simulink model "sampleModel261"  (R2021b)
settings: Solver=VariableStepAuto  StartTime=0.0  StopTime=10.0  RelTol=1e-3
undefined symbols (not defined in the file or in its folder): DiscIntNeverNeededParam
libraries: simulink x6, slpidlib x2
settings Model: Creator=user  LastModifiedBy=user

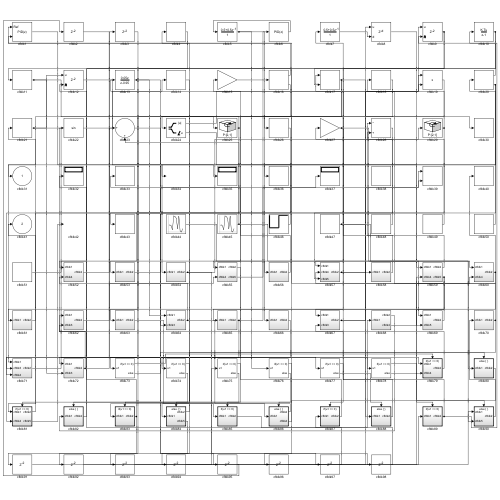
[thumbnail: Simulink's stored preview of the top-level diagram]
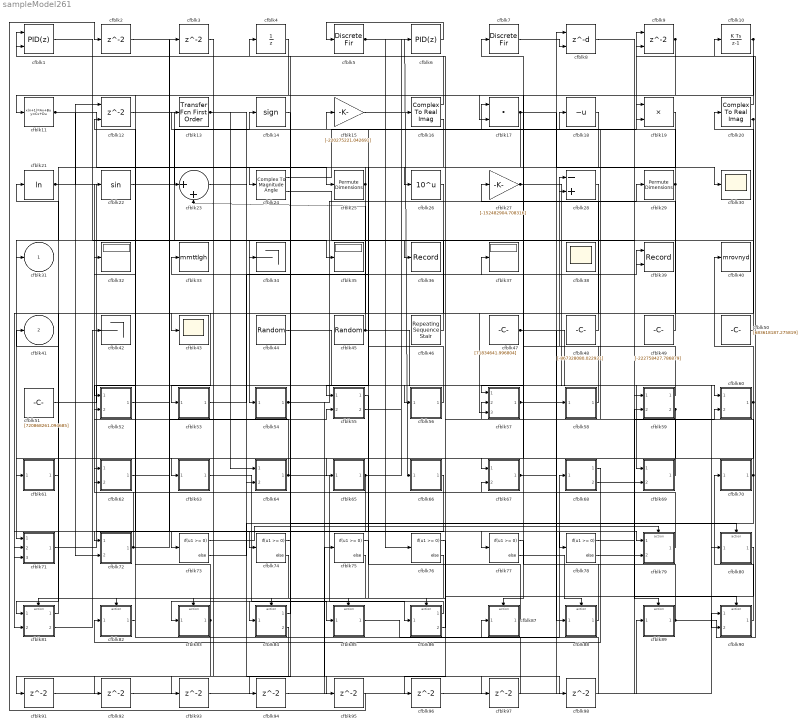
== system sampleModel261 ==
  cfblk1 : slpidlib/PID Controller (2DOF)  Controller=PID  Form=Parallel  TimeDomain=Discrete-time  UseExternalTs=off  SampleTime=1  IntegratorMethod=Forward Euler  FilterMethod=Forward Euler  ControllerParametersSource=internal  P=1  I=1  D=0  UseFilter=on  N=100  b=1  c=1  TunerSelectOption=Transfer Function Based (PID Tuner App)  InitialConditionSource=internal  InitialConditionForIntegrator=0  InitialConditionForFilter=0  DifferentiatorICPrevScaledInput=0  ExternalReset=none  TrackingMode=off  Kt=1  LimitOutput=off  SatLimitsSource=internal  UpperSaturationLimit=inf  LowerSaturationLimit=-inf  LinearizeAsGain=off  AntiWindupMode=none  Kb=1  POutMin=[]  POutMax=[]  IOutMin=[]  IOutMax=[]  DOutMin=[]  DOutMax=[]  NOutMin=[]  NOutMax=[]  bOutMin=[]  bOutMax=[]  cOutMin=[]  cOutMax=[]  SumOutMin=[]  SumOutMax=[]  SaturationOutMin=[]  SaturationOutMax=[]  PParamMin=[]  PParamMax=[]  IParamMin=[]  IParamMax=[]  DParamMin=[]  DParamMax=[]  NParamMin=[]  NParamMax=[]  bParamMin=[]  bParamMax=[]  cParamMin=[]  cParamMax=[]  KbParamMin=[]  KbParamMax=[]  KtParamMin=[]  KtParamMax=[]  KbOutMin=[]  KbOutMax=[]  KtOutMin=[]  KtOutMax=[]  IntegratorOutMin=[]  IntegratorOutMax=[]  FilterOutMin=[]  FilterOutMax=[]  SumI1OutMin=[]  SumI1OutMax=[]  SumI2OutMin=[]  SumI2OutMax=[]  SumI3OutMin=[]  SumI3OutMax=[]  SumI4OutMin=[]  SumI4OutMax=[]  SumDOutMin=[]  SumDOutMax=[]  Sum1OutMin=[]  Sum1OutMax=[]  Sum2OutMin=[]  Sum2OutMax=[]  Sum3OutMin=[]  Sum3OutMax=[]  DifferentiatorOutMin=[]  DifferentiatorOutMax=[]  FilterDiffOutCoefMin=[]  FilterDiffOutCoefMax=[]  ReciprocalOutMin=[]  ReciprocalOutMax=[]  SumDenOutMin=[]  SumDenOutMax=[]  SumNumOutMin=[]  SumNumOutMax=[]  DivideOutMin=[]  DivideOutMax=[]  UdiffTsProdOutMin=[]  UdiffTsProdOutMax=[]  NTsProdOutMin=[]  NTsProdOutMax=[]  UintegralTsProdOutMin=[]  UintegralTsProdOutMax=[]  UngainTsProdOutMin=[]  UngainTsProdOutMax=[]  IntegratorContinuousStateAttributes=''  IntegratorStateMustResolveToSignalObject=off  IntegratorRTWStateStorageClass=Auto  FilterContinuousStateAttributes=''  FilterStateMustResolveToSignalObject=off  FilterRTWStateStorageClass=Auto  ParallelPVariant=InternalParameters  IdealPVariant=Disabled  IVariant=InternalParameters  DVariant=InternalParameters  bVariant=InternalParameters  cVariant=InternalParameters  IntegratorVariant=Discrete  SatVariant=Disabled  AWVariant=Passthrough  PCopyVariant=Disabled  TRVariant=Disabled  FdbkBlocksVariant=Forward  IdealPFdbkVariant=Disabled  SatFdbkVariant=Disabled  DerivativeFilterVariant=ForwardEulerFilter  NVariant=InternalParameters  NCopyVariant=Disabled  FilterICVariant=InternalICsFilter  IntegratorICVariant=InternalICs  ExternalResetVariant=Disabled  TRSumVariant=Passthrough  SumFdbkVariant=Disabled  SumVariant=Sum_PID  TsampFilterVariant=InternalTs  TsampNgainVariant=Passthrough  TsampIntegralVariant=Passthrough  ExternalSaturationOutDataTypeStr=Inherit: Same as second input
      settings: SourceProductBaseCode=SL
  cfblk10 : DiscreteIntegrator  ICPrevOutput=DiscIntNeverNeededParam  ICPrevScaledInput=DiscIntNeverNeededParam
  cfblk11 : DiscreteStateSpace
  cfblk12 : Delay  ShowEnablePort=on  SampleTime=1
      settings: InputPortMap=u0,e6
  cfblk13 : simulink/Discrete/Transfer Fcn First Order  PoleZ=0.95  ICPrevOutput=0.0  DoSatur=off
  cfblk14 : Signum
  cfblk15 : Gain  Gain=[-220275221.042691]
  cfblk16 : ComplexToRealImag
  cfblk17 : DotProduct  InputSameDT=on  OutDataTypeStr=Inherit: Inherit via internal rule
  cfblk18 : UnaryMinus
  cfblk19 : Product
  cfblk{2..3,91..98} (10 alike) : Delay  SampleTime=1
  cfblk20 : ComplexToRealImag
  cfblk21 : Math  Operator=log  SaturateOnIntegerOverflow=on
  cfblk22 : Trigonometry
  cfblk23 : Sum  Inputs=|++
  cfblk24 : ComplexToMagnitudeAngle
  cfblk25 : PermuteDimensions
  cfblk26 : Math  Operator=10^u  SaturateOnIntegerOverflow=on
  cfblk27 : Gain  Gain=[-152482904.708316]
  cfblk28 : Sum  Inputs=-+
  cfblk29 : PermuteDimensions
  cfblk30 : Scope
  cfblk32 : Display
  cfblk33 : ToWorkspace  VariableName=mmttlgh  SaveFormat=Timeseries  SampleTime=-1
  cfblk34 : Terminator
  cfblk35 : Display
  cfblk36 : Record  FileSettingsInternal="{\"entries\":[{\"content\":{\"excelSettings\":{\"content\":{},\"type\":\"Streamout.ExcelSettings\"}},\"type\":\"Streamout.FileSettingStorage\",\"uuid\":\"4783f050-7d98-462b-b792-b8648497e3fe\"}],\"packageUris\":[\"http://schema.mathworks.com/mf0/streamout_blocks/R2020a\"],\"version\":\"1.0\"}"  SignalsInternal="{\"entries\":[{\"content\":{\"signals\":[{\"content\":{\"blockPath\":[\"sampleModel261/cfblk36\"],\"channel\":[],\"dimensions\":[1],\"domain\":\"sampleModel261/cfblk36\",\"lineColor\":\"#ff6929\",\"plots\":[1],\"port\":1,\"sid\":[\"\"],\"signalID\":10888,\"signalName\":\"cfblk20:2\"},\"type\":\"RecordBlkView.Signal\",\"uuid\":\"4df9fe2c-f34f-4dbe-b7be-8e884af156bd\"}]},\"type\":\"RecordBlkView.InputSignals\",\"uuid\":\"7474e692-34f3-44e7-b6b0-6796ef208041\"}],\"packageUris\":[\"http://schema.mathworks.com/mf0/streamout_blocks/R2020a\"],\"version\":\"1.0\"}"  VisualizationBindings="{\"sparklinesplugin\":{\"info\":[{\"bindingParametersList\":[],\"subplotID\":1}]}}"
  cfblk37 : Display
  cfblk38 : Scope
      settings: Floating=on
  cfblk39 : Record  FileSettingsInternal="{\"entries\":[{\"content\":{\"excelSettings\":{\"content\":{},\"type\":\"Streamout.ExcelSettings\"}},\"type\":\"Streamout.FileSettingStorage\",\"uuid\":\"46861a95-7c26-4399-873a-b522a0f094fc\"}],\"packageUris\":[\"http://schema.mathworks.com/mf0/streamout_blocks/R2020a\"],\"version\":\"1.0\"}"  Layout=[1 1]  SignalsInternal="{\"entries\":[{\"content\":{\"signals\":[{\"content\":{\"blockPath\":[\"sampleModel261/cfblk39\"],\"channel\":[],\"dimensions\":[1],\"domain\":\"sampleModel261/cfblk39\",\"lineColor\":\"#a2142f\",\"plots\":[1],\"port\":1,\"sid\":[\"\"],\"signalID\":10892,\"signalName\":\"cfblk53\"},\"type\":\"RecordBlkView.Signal\",\"uuid\":\"985c65e8-5a49-40a9-873e-d05232d7a301\"},{\"content\":{\"blockPath\":[\"sampleModel261/cfblk39\"],\"channel\":[],\"dimensions\":[1],\"domain\":\"sampleModel261/cfblk39\",\"lineColor\":\"#139fff\",\"plots\":[1],\"port\":2,\"sid\":[\"\"],\"signalID\":10896,\"signalName\":\"cfblk67\"},\"type\":\"RecordBlkView.Signal\",\"uuid\":\"3942fdeb-4ef8-4120-b6bd-93e71312b189\"}]},\"type\":\"RecordBlkView.InputSignals\",\"uuid\":\"6ac94be0-a59e-47f5-b2eb-581f409a4b3f\"}],\"packageUris\":[\"http://schema.mathworks.com/mf0/streamout_blocks/R2020a\"],\"version\":\"1.0\"}"  VisualizationBindings="{\"xyplotplugin\":{\"info\":[{\"series\":[{\"bindingParametersList\":[{\"parameter\":\"X-Axis\",\"signalID\":10892,\"signalName\":\"cfblk53\"},{\"parameter\":\"Y-Axis\",\"signalID\":10896,\"signalName\":\"cfblk67\"}],\"seriesID\":48733}],\"subplotID\":1}]}}"  CompatibilityTag=XY
  cfblk4 : UnitDelay  HasFrameUpgradeWarning=on
  cfblk40 : ToWorkspace  VariableName=mrovnyd  SaveFormat=Timeseries  SampleTime=-1
  cfblk42 : Terminator
  cfblk43 : Scope
  cfblk44 : RandomNumber  Mean=[-42971.551268]  Variance=[4965.905583]  Seed=[350835842.000000]  SampleTime=0.1
  cfblk45 : RandomNumber  Mean=[-61962.834245]  Variance=[36079.524142]  Seed=[162837869.000000]  SampleTime=0.1
  cfblk46 : simulink/Sources/Repeating Sequence Stair  OutValues=[-525910598.601651, -330770362.763156]  tsamp=-1  OutMin=[]  OutMax=[]  OutDataTypeStr=double  OutputDataTypeScalingMode=double  OutDataType=fixdt(0,8)  ConRadixGroup=Best Precision: Vector-wise  OutScaling=2^-12
  cfblk47 : Constant  Value=[71834641.996804]  SampleTime=1
  cfblk48 : Constant  Value=[-867328080.022931]  SampleTime=1
  cfblk49 : Constant  Value=[-222758427.786879]  SampleTime=1
  cfblk5 : DiscreteFir  SampleTime=1
  cfblk50 : Constant  Value=[683618187.275819]  SampleTime=1
  cfblk51 : Constant  Value=[720868261.094685]  SampleTime=1
  cfblk52 : Subsystem
  cfblk53 : Subsystem
  cfblk54 : Subsystem
  cfblk55 : Subsystem
  cfblk56 : Subsystem
  cfblk57 : Subsystem
  cfblk58 : Subsystem
  cfblk59 : Subsystem
  cfblk6 : slpidlib/PID Controller  Controller=PID  Form=Parallel  TimeDomain=Discrete-time  UseExternalTs=off  SampleTime=1  IntegratorMethod=Forward Euler  FilterMethod=Forward Euler  ControllerParametersSource=internal  P=1  I=1  D=0  UseFilter=on  N=100  TunerSelectOption=Transfer Function Based (PID Tuner App)  InitialConditionSource=internal  InitialConditionForIntegrator=0  InitialConditionForFilter=0  DifferentiatorICPrevScaledInput=0  ExternalReset=none  TrackingMode=off  Kt=1  LimitOutput=off  SatLimitsSource=internal  UpperSaturationLimit=inf  LowerSaturationLimit=-inf  LinearizeAsGain=off  AntiWindupMode=none  Kb=1  POutMin=[]  POutMax=[]  IOutMin=[]  IOutMax=[]  DOutMin=[]  DOutMax=[]  NOutMin=[]  NOutMax=[]  SumOutMin=[]  SumOutMax=[]  SaturationOutMin=[]  SaturationOutMax=[]  PParamMin=[]  PParamMax=[]  IParamMin=[]  IParamMax=[]  DParamMin=[]  DParamMax=[]  NParamMin=[]  NParamMax=[]  KbParamMin=[]  KbParamMax=[]  KtParamMin=[]  KtParamMax=[]  KbOutMin=[]  KbOutMax=[]  KtOutMin=[]  KtOutMax=[]  IntegratorOutMin=[]  IntegratorOutMax=[]  FilterOutMin=[]  FilterOutMax=[]  SumI1OutMin=[]  SumI1OutMax=[]  SumI2OutMin=[]  SumI2OutMax=[]  SumI3OutMin=[]  SumI3OutMax=[]  SumI4OutMin=[]  SumI4OutMax=[]  SumDOutMin=[]  SumDOutMax=[]  DifferentiatorOutMin=[]  DifferentiatorOutMax=[]  FilterDiffOutCoefMin=[]  FilterDiffOutCoefMax=[]  ReciprocalOutMin=[]  ReciprocalOutMax=[]  SumDenOutMin=[]  SumDenOutMax=[]  SumNumOutMin=[]  SumNumOutMax=[]  DivideOutMin=[]  DivideOutMax=[]  UdiffTsProdOutMin=[]  UdiffTsProdOutMax=[]  NTsProdOutMin=[]  NTsProdOutMax=[]  UintegralTsProdOutMin=[]  UintegralTsProdOutMax=[]  UngainTsProdOutMin=[]  UngainTsProdOutMax=[]  IntegratorContinuousStateAttributes=''  IntegratorStateMustResolveToSignalObject=off  IntegratorRTWStateStorageClass=Auto  FilterContinuousStateAttributes=''  FilterStateMustResolveToSignalObject=off  FilterRTWStateStorageClass=Auto  ParallelPVariant=InternalParameters  IdealPVariant=Disabled  IVariant=InternalParameters  DVariant=InternalParameters  IntegratorVariant=Discrete  SatVariant=Disabled  AWVariant=Passthrough  PCopyVariant=Disabled  TRVariant=Disabled  FdbkBlocksVariant=Forward  IdealPFdbkVariant=Disabled  SatFdbkVariant=Disabled  DerivativeFilterVariant=ForwardEulerFilter  NVariant=InternalParameters  NCopyVariant=Disabled  FilterICVariant=InternalICsFilter  IntegratorICVariant=InternalICs  ExternalResetVariant=Disabled  TRSumVariant=Passthrough  SumFdbkVariant=Disabled  SumVariant=Sum_PID  TsampFilterVariant=InternalTs  TsampNgainVariant=Passthrough  TsampIntegralVariant=Passthrough  ExternalSaturationOutDataTypeStr=Inherit: Same as second input
  cfblk60 : Subsystem
  cfblk61 : Subsystem
  cfblk62 : Subsystem
  cfblk63 : Subsystem
  cfblk64 : Subsystem
  cfblk65 : Subsystem
  cfblk66 : Subsystem
  cfblk67 : Subsystem
  cfblk68 : Subsystem
  cfblk69 : Subsystem
  cfblk7 : DiscreteFir  SampleTime=1
  cfblk70 : Subsystem
  cfblk71 : Subsystem
  cfblk72 : Subsystem
  cfblk{73..78} (6 alike) : If  IfExpression=u1 >= 0  SampleTime=1
  cfblk79 : Subsystem  TreatAsAtomicUnit=on
  cfblk8 : Delay  DelayLengthSource=Input port  SampleTime=1
      settings: InputPortMap=u0,p1
  cfblk80 : Subsystem  TreatAsAtomicUnit=on
  cfblk81 : Subsystem  TreatAsAtomicUnit=on
  cfblk82 : Subsystem  TreatAsAtomicUnit=on
  cfblk83 : Subsystem  TreatAsAtomicUnit=on
  cfblk84 : Subsystem  TreatAsAtomicUnit=on
  cfblk85 : Subsystem  TreatAsAtomicUnit=on
  cfblk86 : Subsystem  TreatAsAtomicUnit=on
  cfblk87 : Subsystem  TreatAsAtomicUnit=on
  cfblk88 : Subsystem  TreatAsAtomicUnit=on
  cfblk89 : Subsystem  TreatAsAtomicUnit=on
  cfblk9 : Delay  ShowEnablePort=on  SampleTime=1
      settings: InputPortMap=u0,e6
  cfblk90 : Subsystem  TreatAsAtomicUnit=on
  cfblk31 : Outport
  cfblk41 : Outport  Port=2
  wires:
  cfblk64/1(cfblk2) -> cfblk86/1(cfblk1), cfblk52/2(cfblk4)
  cfblk87/1(cfblk2) -> cfblk33/1
  cfblk46/1 -> cfblk71/1(cfblk1)
  cfblk12/1 -> cfblk54/1(cfblk1)
  cfblk69/1(cfblk2) -> cfblk11/1
  cfblk85/1(cfblk2) -> cfblk68/1(cfblk1)
  cfblk68/1(cfblk2) -> cfblk82/1(cfblk1)
  cfblk47/1 -> cfblk88/1(cfblk1), cfblk80/1(cfblk1)
  cfblk5/1 -> cfblk66/1(cfblk1), cfblk76/1
  cfblk45/1 -> cfblk69/1(cfblk1), cfblk23/2
  cfblk49/1 -> cfblk28/1
  cfblk81/1(cfblk2) -> cfblk41/1
  cfblk29/1 -> cfblk13/1, cfblk71/3(cfblk4)
  cfblk54/1(cfblk2) -> cfblk29/1, cfblk98/1
  cfblk6/1 -> cfblk5/1
  cfblk67/1(cfblk2) -> cfblk58/1(cfblk1), cfblk39/2
  cfblk89/1(cfblk2) -> cfblk9/1, cfblk67/2(cfblk3)
  cfblk27/1 -> cfblk90/2(cfblk5), cfblk67/1(cfblk1)
  cfblk60/1(cfblk2) -> cfblk40/1, cfblk65/1(cfblk1), cfblk57/2(cfblk4)
  cfblk19/1 -> cfblk26/1
  cfblk44/1 -> cfblk60/1(cfblk1)
  cfblk61/1(cfblk2) -> cfblk21/1
  cfblk62/1(cfblk2) -> cfblk3/1
  cfblk20/1 -> cfblk10/1
  cfblk48/1 -> cfblk27/1
  cfblk55/1(cfblk2) -> cfblk71/2(cfblk3)
  cfblk51/1 -> cfblk56/1(cfblk1)
  cfblk21/1 -> cfblk78/1, cfblk12/1
  cfblk65/1(cfblk2) -> cfblk37/1, cfblk81/2(cfblk4)
  cfblk55/2(cfblk5) -> cfblk16/1
  cfblk2/1 -> cfblk77/1
  cfblk90/1(cfblk2) -> cfblk70/1(cfblk1)
  cfblk4/1 -> cfblk43/1
  cfblk63/1(cfblk2) -> cfblk85/1(cfblk1)
  cfblk66/1(cfblk2) -> cfblk74/1
  cfblk24/1 -> cfblk9/2
  cfblk53/1(cfblk2) -> cfblk39/1
  cfblk22/1 -> cfblk14/1
  cfblk71/1(cfblk2) -> cfblk79/1(cfblk1)
  cfblk88/1(cfblk2) -> cfblk7/1
  cfblk11/1 -> cfblk25/1, cfblk72/2(cfblk3)
  cfblk18/1 -> cfblk31/1
  cfblk56/1(cfblk2) -> cfblk15/1
  cfblk86/1(cfblk2) -> cfblk83/1(cfblk1)
  cfblk28/1 -> cfblk53/1(cfblk1)
  cfblk25/1 -> cfblk63/1(cfblk1), cfblk24/1
  cfblk79/1(cfblk2) -> cfblk22/1
  cfblk16/1 -> cfblk1/1
  cfblk70/1(cfblk2) -> cfblk18/1, cfblk94/1
  cfblk59/1(cfblk2) -> cfblk28/2
  cfblk52/1(cfblk2) -> cfblk23/1
  cfblk84/1(cfblk2) -> cfblk4/1
  cfblk26/1 -> cfblk81/1(cfblk1)
  cfblk7/1 -> cfblk8/2
  cfblk9/1 -> cfblk57/1(cfblk1), cfblk17/2
  cfblk10/1 -> cfblk52/1(cfblk1), cfblk72/1(cfblk1)
  cfblk14/1 -> cfblk84/1(cfblk1)
  cfblk83/1(cfblk2) -> cfblk62/2(cfblk3), cfblk91/1
  cfblk1/1 -> cfblk35/1
  cfblk58/1(cfblk2) -> cfblk17/1
  cfblk16/2 -> cfblk73/1
  cfblk82/1(cfblk2) -> cfblk32/1
  cfblk24/2 -> cfblk79/2(cfblk4)
  cfblk72/1(cfblk2) -> cfblk62/1(cfblk1), cfblk55/2(cfblk4)
  cfblk8/1 -> cfblk59/1(cfblk1)
  cfblk86/2(cfblk4) -> cfblk1/2
  cfblk68/2(cfblk4) -> cfblk60/2(cfblk4)
  cfblk81/2(cfblk5) -> cfblk42/1
  cfblk20/2 -> cfblk36/1, cfblk34/1, cfblk57/3(cfblk5)
  cfblk59/2(cfblk5) -> cfblk61/1(cfblk1), cfblk69/2(cfblk5)
  cfblk13/1 -> cfblk64/1(cfblk1), cfblk97/1
  cfblk50/1 -> cfblk20/1
  cfblk15/1 -> cfblk6/1
  cfblk17/1 -> cfblk30/1, cfblk64/2(cfblk3), cfblk55/1(cfblk1)
  cfblk57/1(cfblk2) -> cfblk19/1, cfblk19/2
  cfblk73/1 -> cfblk79/Action
  cfblk73/2 -> cfblk80/Action
  cfblk74/1 -> cfblk81/Action
  cfblk74/2 -> cfblk82/Action
  cfblk75/1 -> cfblk83/Action
  cfblk75/2 -> cfblk84/Action
  cfblk76/1 -> cfblk85/Action
  cfblk76/2 -> cfblk86/Action
  cfblk77/1 -> cfblk87/Action
  cfblk77/2 -> cfblk88/Action
  cfblk78/1 -> cfblk89/Action
  cfblk78/2 -> cfblk90/Action
  cfblk91/1 -> cfblk75/1
  cfblk84/2(cfblk5) -> cfblk92/1
  cfblk92/1 -> cfblk59/2(cfblk4)
  cfblk3/1 -> cfblk93/1
  cfblk93/1 -> cfblk90/1(cfblk1)
  cfblk94/1 -> cfblk89/1(cfblk1)
  cfblk23/1 -> cfblk95/1
  cfblk95/1 -> cfblk2/1
  cfblk80/1(cfblk2) -> cfblk96/1
  cfblk96/1 -> cfblk8/1
  cfblk97/1 -> cfblk87/1(cfblk1)
  cfblk98/1 -> cfblk12/2

== system sampleModel261/cfblk52 ==
  cfblk1 : Inport
  cfblk4 : Inport  Port=2
  cfblk3 : Gain  Gain=[-502459091.034332]
  cfblk2 : Outport
  wires:
  cfblk3/1 -> cfblk2/1
  cfblk1/1 -> cfblk3/1

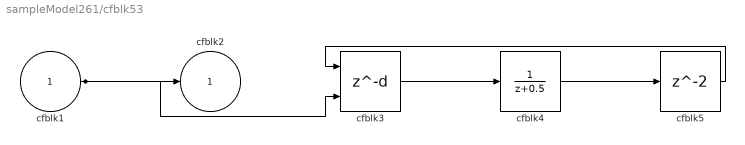
== system sampleModel261/cfblk53 ==
  cfblk1 : Inport
  cfblk3 : Delay  DelayLengthSource=Input port  SampleTime=1
      settings: InputPortMap=u0,p1
  cfblk4 : DiscreteTransferFcn  SampleTime=1
  cfblk5 : Delay  SampleTime=1
  cfblk2 : Outport
  wires:
  cfblk1/1 -> cfblk2/1, cfblk3/2
  cfblk3/1 -> cfblk4/1
  cfblk4/1 -> cfblk5/1
  cfblk5/1 -> cfblk3/1

== system sampleModel261/cfblk54 ==
  cfblk1 : Inport
  cfblk3 : Constant  Value=[-375122664.981902]  SampleTime=1
  cfblk2 : Outport
  wires:
  cfblk3/1 -> cfblk2/1

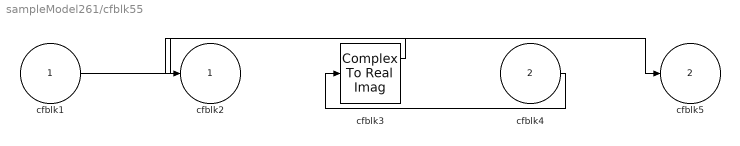
== system sampleModel261/cfblk55 ==
  cfblk1 : Inport
  cfblk4 : Inport  Port=2
  cfblk3 : ComplexToRealImag
  cfblk2 : Outport
  cfblk5 : Outport  Port=2
  wires:
  cfblk1/1 -> cfblk5/1
  cfblk4/1 -> cfblk3/1
  cfblk3/1 -> cfblk2/1

== system sampleModel261/cfblk56 ==
  cfblk1 : Inport
  cfblk3 : simulink/Discrete/Tapped Delay  vinit=0.0  samptime=-1  NumDelays=1  DelayOrder=Oldest  includeCurrent=off
  cfblk2 : Outport
  wires:
  cfblk1/1 -> cfblk3/1
  cfblk3/1 -> cfblk2/1

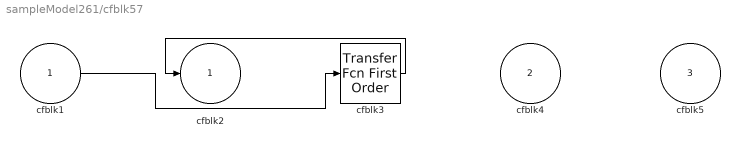
== system sampleModel261/cfblk57 ==
  cfblk1 : Inport
  cfblk4 : Inport  Port=2
  cfblk5 : Inport  Port=3
  cfblk3 : simulink/Discrete/Transfer Fcn First Order  PoleZ=0.95  ICPrevOutput=0.0  DoSatur=off
  cfblk2 : Outport
  wires:
  cfblk3/1 -> cfblk2/1
  cfblk1/1 -> cfblk3/1

== system sampleModel261/cfblk58 ==
  cfblk1 : Inport
  cfblk3 : Constant  Value=[649967012.851321]  SampleTime=1
  cfblk2 : Outport
  wires:
  cfblk3/1 -> cfblk2/1

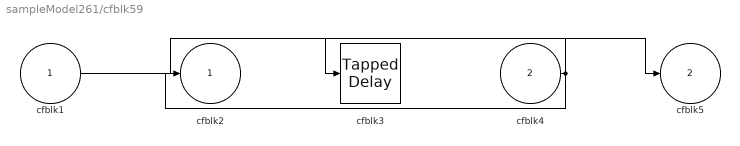
== system sampleModel261/cfblk59 ==
  cfblk1 : Inport
  cfblk4 : Inport  Port=2
  cfblk3 : simulink/Discrete/Tapped Delay  vinit=0.0  samptime=-1  NumDelays=1  DelayOrder=Oldest  includeCurrent=off
  cfblk2 : Outport
  cfblk5 : Outport  Port=2
  wires:
  cfblk1/1 -> cfblk5/1
  cfblk4/1 -> cfblk2/1, cfblk3/1

== system sampleModel261/cfblk60 ==
  cfblk1 : Inport
  cfblk4 : Inport  Port=2
  cfblk3 : DiscreteFilter  SampleTime=1
  cfblk2 : Outport
  wires:
  cfblk4/1 -> cfblk3/1
  cfblk3/1 -> cfblk2/1

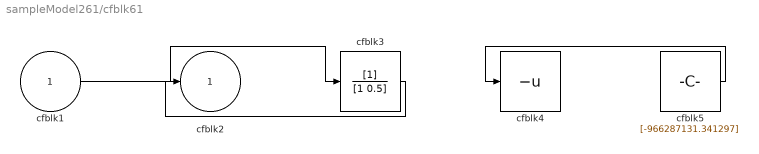
== system sampleModel261/cfblk61 ==
  cfblk1 : Inport
  cfblk3 : DiscreteFilter  SampleTime=1
  cfblk4 : UnaryMinus
  cfblk5 : Constant  Value=[-966287131.341297]  SampleTime=1
  cfblk2 : Outport
  wires:
  cfblk1/1 -> cfblk3/1
  cfblk3/1 -> cfblk2/1
  cfblk5/1 -> cfblk4/1

== system sampleModel261/cfblk62 ==
  cfblk1 : Inport
  cfblk3 : Inport  Port=2
  cfblk2 : Outport
  wires:
  cfblk3/1 -> cfblk2/1

== system sampleModel261/cfblk63 ==
  cfblk1 : Inport
  cfblk3 : Constant  Value=[706782325.083097]  SampleTime=1
  cfblk2 : Outport
  wires:
  cfblk3/1 -> cfblk2/1

== system sampleModel261/cfblk64 ==
  cfblk1 : Inport
  cfblk3 : Inport  Port=2
  cfblk2 : Outport
  wires:
  cfblk3/1 -> cfblk2/1

== system sampleModel261/cfblk65 ==
  cfblk1 : Inport
  cfblk3 : Assignment  DiagnosticForDimensions=Warning  IndexOptions=Index vector (dialog)  Indices=1  OutputSizes=1
  cfblk2 : Outport
  wires:
  cfblk1/1 -> cfblk3/1, cfblk3/2
  cfblk3/1 -> cfblk2/1

== system sampleModel261/cfblk66 ==
  cfblk1 : Inport
  cfblk3 : Constant  Value=[-774883804.689383]  SampleTime=1
  cfblk4 : Constant  Value=[-642052171.851356]  SampleTime=1
  cfblk2 : Outport
  wires:
  cfblk3/1 -> cfblk2/1

== system sampleModel261/cfblk67 ==
  cfblk1 : Inport
  cfblk3 : Inport  Port=2
  cfblk2 : Outport
  wires:
  cfblk3/1 -> cfblk2/1

== system sampleModel261/cfblk68 ==
  cfblk1 : Inport
  cfblk3 : DiscreteZeroPole  Poles=[0 0.5]  Gain=1
  cfblk2 : Outport
  cfblk4 : Outport  Port=2
  wires:
  cfblk1/1 -> cfblk4/1, cfblk3/1
  cfblk3/1 -> cfblk2/1

== system sampleModel261/cfblk69 ==
  cfblk1 : Inport
  cfblk5 : Inport  Port=2
  cfblk3 : Product  Inputs=*
  cfblk4 : Constant  Value=[177762954.511539]  SampleTime=1
  cfblk2 : Outport
  wires:
  cfblk4/1 -> cfblk2/1
  cfblk1/1 -> cfblk3/1

== system sampleModel261/cfblk70 ==
  cfblk1 : Inport
  cfblk3 : UnaryMinus
  cfblk2 : Outport
  wires:
  cfblk3/1 -> cfblk2/1
  cfblk1/1 -> cfblk3/1

== system sampleModel261/cfblk71 ==
  cfblk1 : Inport
  cfblk3 : Inport  Port=2
  cfblk4 : Inport  Port=3
  cfblk2 : Outport
  wires:
  cfblk4/1 -> cfblk2/1

== system sampleModel261/cfblk72 ==
  cfblk1 : Inport
  cfblk3 : Inport  Port=2
  cfblk2 : Outport
  wires:
  cfblk3/1 -> cfblk2/1

== system sampleModel261/cfblk79 ==
  cfblk1 : Inport
  cfblk4 : Inport  Port=2
  Action Port : ActionPort  ActionPortLabel=if(u1 >= 0)
  cfblk3 : DiscreteTransferFcn
  cfblk2 : Outport
  wires:
  cfblk4/1 -> cfblk2/1
  cfblk1/1 -> cfblk3/1

== system sampleModel261/cfblk80 ==
  cfblk1 : Inport
  Action Port : ActionPort  ActionPortLabel=else
  cfblk3 : Reshape
  cfblk4 : Product  Inputs=*
  cfblk2 : Outport
  wires:
  cfblk1/1 -> cfblk4/1
  cfblk4/1 -> cfblk3/1
  cfblk3/1 -> cfblk2/1

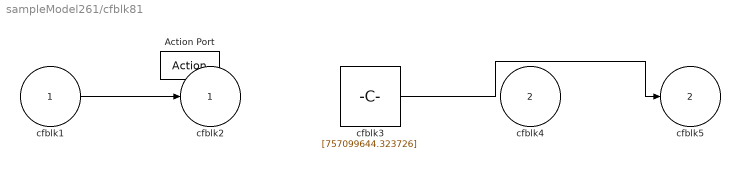
== system sampleModel261/cfblk81 ==
  cfblk1 : Inport
  cfblk4 : Inport  Port=2
  Action Port : ActionPort  ActionPortLabel=if(u1 >= 0)
  cfblk3 : Constant  Value=[757099644.323726]  SampleTime=1
  cfblk2 : Outport
  cfblk5 : Outport  Port=2
  wires:
  cfblk3/1 -> cfblk5/1
  cfblk1/1 -> cfblk2/1

== system sampleModel261/cfblk82 ==
  cfblk1 : Inport
  Action Port : ActionPort  ActionPortLabel=else
  cfblk3 : DotProduct  InputSameDT=on  OutDataTypeStr=Inherit: Inherit via internal rule
  cfblk2 : Outport
  wires:
  cfblk1/1 -> cfblk2/1, cfblk3/1, cfblk3/2

== system sampleModel261/cfblk83 ==
  cfblk1 : Inport
  Action Port : ActionPort  ActionPortLabel=if(u1 >= 0)
  cfblk3 : Rounding
  cfblk4 : Constant  Value=[-338983970.118135]  SampleTime=1
  cfblk2 : Outport
  wires:
  cfblk4/1 -> cfblk3/1
  cfblk3/1 -> cfblk2/1

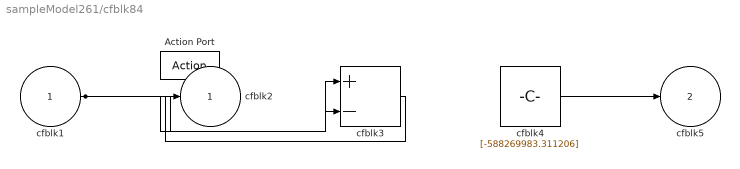
== system sampleModel261/cfblk84 ==
  cfblk1 : Inport
  Action Port : ActionPort  ActionPortLabel=else
  cfblk3 : Sum  Inputs=+-
  cfblk4 : Constant  Value=[-588269983.311206]  SampleTime=1
  cfblk2 : Outport
  cfblk5 : Outport  Port=2
  wires:
  cfblk4/1 -> cfblk5/1
  cfblk1/1 -> cfblk3/1, cfblk3/2
  cfblk3/1 -> cfblk2/1

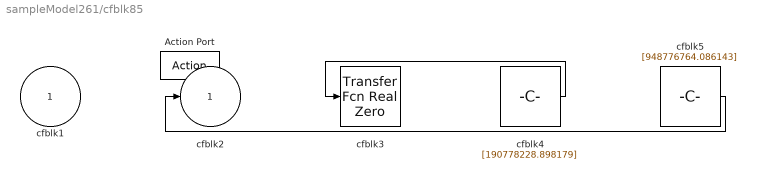
== system sampleModel261/cfblk85 ==
  cfblk1 : Inport
  Action Port : ActionPort  ActionPortLabel=if(u1 >= 0)
  cfblk3 : simulink/Discrete/Transfer Fcn Real Zero  ZeroZ=0.75  ICPrevInput=0.0  DoSatur=off
      settings: SourceProductBaseCode=SL
  cfblk4 : Constant  Value=[190778228.898179]  SampleTime=1
  cfblk5 : Constant  Value=[948776764.086143]  SampleTime=1
  cfblk2 : Outport
  wires:
  cfblk5/1 -> cfblk2/1
  cfblk4/1 -> cfblk3/1

== system sampleModel261/cfblk86 ==
  cfblk1 : Inport
  Action Port : ActionPort  ActionPortLabel=else
  cfblk3 : Reshape
  cfblk2 : Outport
  cfblk4 : Outport  Port=2
  wires:
  cfblk1/1 -> cfblk2/1, cfblk3/1
  cfblk3/1 -> cfblk4/1

== system sampleModel261/cfblk87 ==
  cfblk1 : Inport
  Action Port : ActionPort  ActionPortLabel=if(u1 >= 0)
  cfblk3 : Product  Inputs=*
  cfblk2 : Outport
  wires:
  cfblk1/1 -> cfblk3/1
  cfblk3/1 -> cfblk2/1

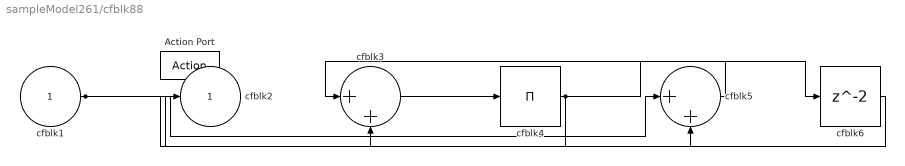
== system sampleModel261/cfblk88 ==
  cfblk1 : Inport
  Action Port : ActionPort  ActionPortLabel=else
  cfblk3 : Sum  Inputs=|++
  cfblk4 : Product  Inputs=*
  cfblk5 : Sum  Inputs=|++
  cfblk6 : Delay
  cfblk2 : Outport
  wires:
  cfblk1/1 -> cfblk5/1, cfblk5/2
  cfblk5/1 -> cfblk3/1
  cfblk4/1 -> cfblk2/1, cfblk6/1
  cfblk3/1 -> cfblk4/1
  cfblk6/1 -> cfblk3/2

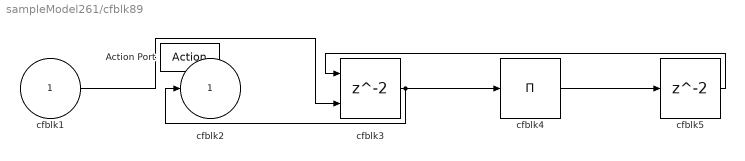
== system sampleModel261/cfblk89 ==
  cfblk1 : Inport
  Action Port : ActionPort  ActionPortLabel=if(u1 >= 0)
  cfblk3 : Delay  ShowEnablePort=on
      settings: InputPortMap=u0,e6
  cfblk4 : Product  Inputs=*
  cfblk5 : Delay
  cfblk2 : Outport
  wires:
  cfblk3/1 -> cfblk2/1, cfblk4/1
  cfblk1/1 -> cfblk3/2
  cfblk4/1 -> cfblk5/1
  cfblk5/1 -> cfblk3/1

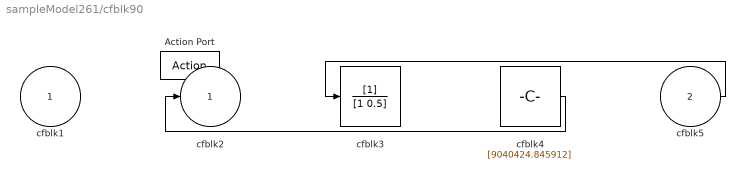
== system sampleModel261/cfblk90 ==
  cfblk1 : Inport
  cfblk5 : Inport  Port=2
  Action Port : ActionPort  ActionPortLabel=else
  cfblk3 : DiscreteFilter
  cfblk4 : Constant  Value=[9040424.845912]  SampleTime=1
  cfblk2 : Outport
  wires:
  cfblk4/1 -> cfblk2/1
  cfblk5/1 -> cfblk3/1
